simulink model "System_HybridMotorcycle_v2"  (R2013a)
settings: Solver=ode15s  StartTime=0.0  StopTime=500  RelTol=1e-3
values from neighbouring files (symbols this model uses):
  HEV_Param =     [Initialization_v2.mat]
  Speed = SpeedMatrix(i)    [Troubleshooting_Engine_v2_Script1.m]
undefined symbols (not defined in the file or in its folder): Acid, Kt, Kt_Temps, Lead, sigbuilder_block, theta_f, theta_init
libraries: fl_lib x56, nesl_utility x30, sdl_lib x6, LeadAcidBattery_lib x6, simulink x1, electricdrivelib x1, elec_lib x1
(part 1 of 2)
settings Model: Creator=Raymond  LastModifiedBy=Raymond

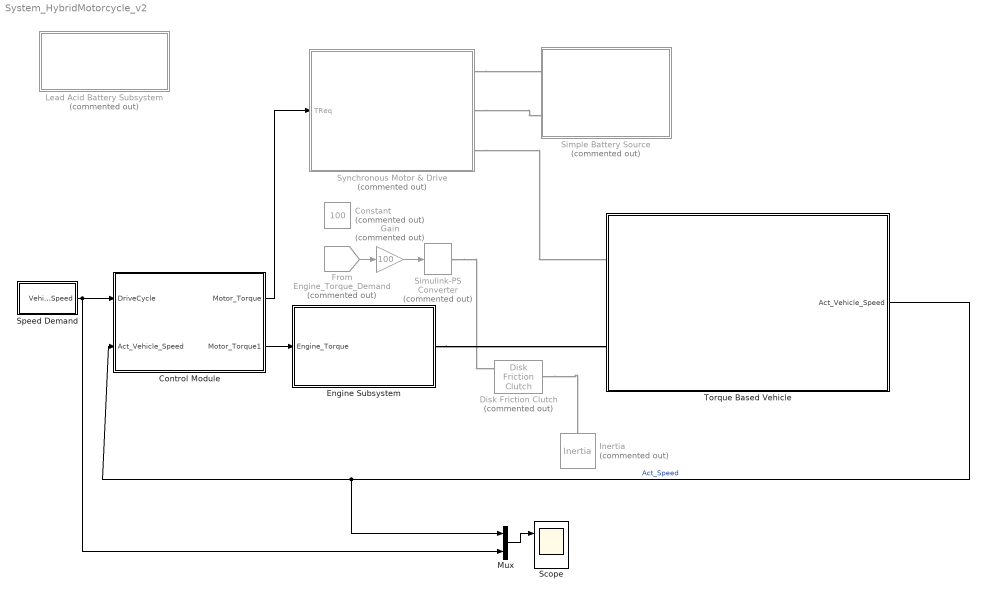
== system System_HybridMotorcycle_v2 ==
  Constant : Constant  Commented=on  Value=100
  Control Module : Subsystem
  Disk Friction Clutch : sdl_lib/Clutches/Disk Friction Clutch  Commented=on  geometry_model=1  r_eff=130 mm  d_o=150 mm  d_i=100 mm  nS=4  piston_area=0.001 m^2  friction_model=1  mu_coulomb=0.3  mu_w_vector=[ 0 0.1 0.2 0.3 0.4 0.5 1 2 5 10 100 1000 ] rad/s  mu_coulomb_vector=[ 0.29 0.28 0.26 0.22 0.21 0.2 0.2 0.19 0.19 0.19 0.19 0.19 ]  mu_interp_method=1  mu_extrap_method=1  mu_static=0.35  d_f=1  w_tol=0.001 rad/s  pressure_min=0.1 Pa  mu_visc=0 N*m/(rad/s)  initial_state_locked=0  LocalVarLogging=[]
  Engine Subsystem : Subsystem
  From : From  Commented=on  GotoTag=Engine_Torque_Demand  TagVisibility=global
  Gain : Gain  Commented=on  Gain=100
  Inertia : fl_lib/Mechanical/Rotational Elements/Inertia  Commented=on  inertia=0.01 kg*m^2  initial_velocity=0 rad/s  t_Log=off  LocalVarNames=|t  LocalVarDescs=|t  LocalVarLogging=0
  Lead Acid Battery Subsystem : Subsystem  Commented=on
  Mux : Mux  Inputs=2
  Scope : Scope  NumInputPorts=2
      settings: YMin=-2.5~0  YMax=50~50  SaveName=ScopeData2
  Simple Battery Source : Subsystem  Commented=on
      mask Display: disp('Simple Battery')
  Simulink-PS Converter : nesl_utility/Simulink-PS Converter  Commented=on  PhysicalDomain=network_engine_domain  SubClassName=ps_input  LeftPortType=input  RightPortType=output  PseudoPeriodic=off  Frequencies=[]  NoiseDistribution=none  NoiseParameters=[]  Unit=1  AffineConversion=off  InputFiltering=off  SimscapeFilterOrder=1  InputFilterTimeConstant=0.001  UdotUserProvided=1
  Speed Demand : Subsystem
      mask Display: disp('DriveCycle')
  Synchronous Motor & Drive : Subsystem  Commented=on
      mask Display:
      | image(imread('HEV_System_Motor_IMAGE.jpg'));
      | port_label('input',1,'T_Req');
      | port_label('RConn',1,'+');
      | port_label('RConn',2,'-');
      | port_label('RConn',3,'Shaft');
  "Torque Based Vehicle " : Subsystem
  wires:
  Speed Demand/1(VehicleSpeed) -> Mux/2, Control Module/1(DriveCycle)
  Control Module/1(Motor_Torque) -> Synchronous Motor & Drive/1(TReq)
  Control Module/2(Motor_Torque1) -> Engine Subsystem/1(Engine_Torque)
  "Torque Based Vehicle "/1(Act_Vehicle_Speed) -> Mux/1, Control Module/2(Act_Vehicle_Speed)  "Act_Speed"
  From/1 -> Gain/1
  Gain/1 -> Simulink-PS Converter/1
  Mux/1 -> Scope/1
  connections:
  Synchronous Motor & Drive/RConn2 -- Simple Battery Source/LConn2
  Synchronous Motor & Drive/RConn1 -- Simple Battery Source/LConn1
  Synchronous Motor & Drive/RConn3 -- "Torque Based Vehicle "/LConn1
  Simulink-PS Converter/RConn1 -- Disk Friction Clutch/LConn1
  Disk Friction Clutch/RConn1 -- Inertia/LConn1
  Engine Subsystem/RConn1 -- "Torque Based Vehicle "/LConn2

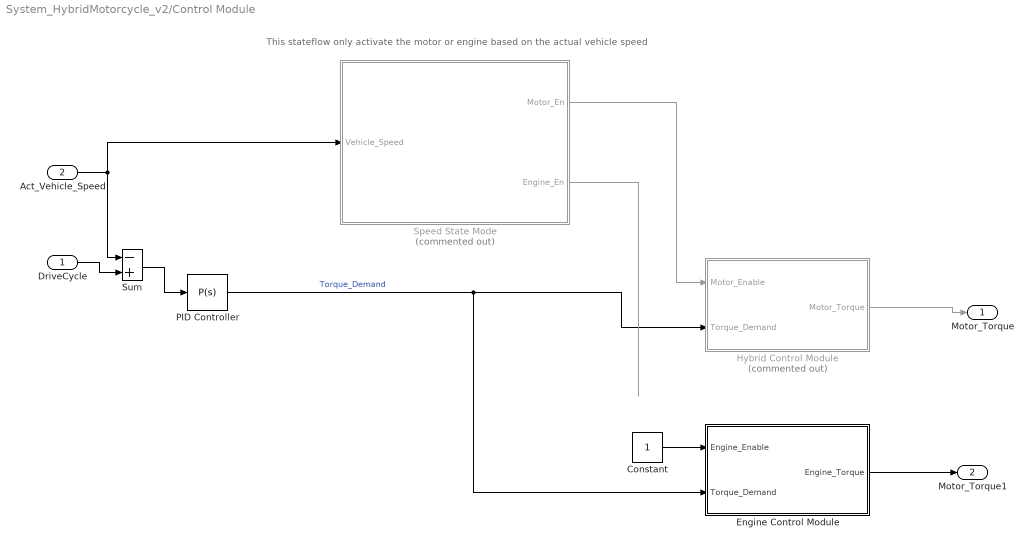
== system System_HybridMotorcycle_v2/Control Module ==
  note: This stateflow only activate the motor or engine
      | based on the actual vehicle speed
  DriveCycle : Inport
  Act_Vehicle_Speed : Inport  Port=2
  Constant : Constant
  Engine Control Module : Subsystem
  Hybrid Control Module : Subsystem  Commented=on
  PID Controller : simulink/Continuous/PID Controller  Controller=P  TimeDomain=Continuous-time  SampleTime=1  IntegratorMethod=Forward Euler  FilterMethod=Forward Euler  Form=Parallel  P=100  I=0  D=0  N=0  InitialConditionSource=internal  InitialConditionForIntegrator=0  InitialConditionForFilter=0  ExternalReset=none  LimitOutput=off  UpperSaturationLimit=inf  LowerSaturationLimit=-inf  LinearizeAsGain=on  AntiWindupMode=none  Kb=1  TrackingMode=off  Kt=1  PParamMin=[]  PParamMax=[]  IParamMin=[]  IParamMax=[]  DParamMin=[]  DParamMax=[]  NParamMin=[]  NParamMax=[]  KbParamMin=[]  KbParamMax=[]  KtParamMin=[]  KtParamMax=[]  POutMin=[]  POutMax=[]  IOutMin=[]  IOutMax=[]  DOutMin=[]  DOutMax=[]  NOutMin=[]  NOutMax=[]  KbOutMin=[]  KbOutMax=[]  KtOutMin=[]  KtOutMax=[]  IntegratorOutMin=[]  IntegratorOutMax=[]  FilterOutMin=[]  FilterOutMax=[]  SumOutMin=[]  SumOutMax=[]  SumI1OutMin=[]  SumI1OutMax=[]  SumI2OutMin=[]  SumI2OutMax=[]  SumI3OutMin=[]  SumI3OutMax=[]  SumDOutMin=[]  SumDOutMax=[]  SaturationOutMin=[]  SaturationOutMax=[]  IntegratorContinuousStateAttributes=''  IntegratorStateMustResolveToSignalObject=off  IntegratorRTWStateStorageClass=Auto  FilterContinuousStateAttributes=''  FilterStateMustResolveToSignalObject=off  FilterRTWStateStorageClass=Auto
  Speed State Mode : Stateflow chart  Commented=on  TreatAsAtomicUnit=on
  Sum : Sum  Inputs=-+
  Motor_Torque : Outport
  Motor_Torque1 : Outport  Port=2
  wires:
  Sum/1 -> PID Controller/1
  PID Controller/1 -> Engine Control Module/2(Torque_Demand), Hybrid Control Module/2(Torque_Demand)  "Torque_Demand"
  Speed State Mode/2(Engine_En) -> ?
  Speed State Mode/1(Motor_En) -> Hybrid Control Module/1(Motor_Enable)
  Hybrid Control Module/1(Motor_Torque) -> Motor_Torque/1
  Engine Control Module/1(Engine_Torque) -> Motor_Torque1/1
  DriveCycle/1 -> Sum/2
  Act_Vehicle_Speed/1 -> Speed State Mode/1(Vehicle_Speed), Sum/1
  Constant/1 -> Engine Control Module/1(Engine_Enable)

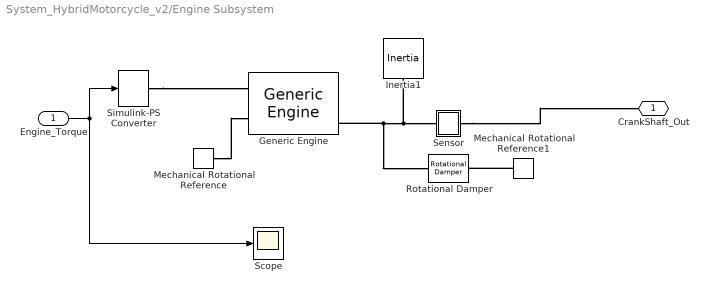
== system System_HybridMotorcycle_v2/Engine Subsystem ==
  Engine_Torque : Inport
  Generic Engine : sdl_lib/Engines/Generic Engine  model_parameterization=1  engine_type=1  P_max=8300 W  w_P_max=8500 rpm  w_max=9000 rpm  w_min=500 rpm  w_tab=[ 500 1000 2e+3 3e+3 4e+3 5e+3 6e+3 7e+3 ] rpm  trq_tab=[ 380 380 380 380 350 280 200 80 ] N*m  pwr_tab=[ 2e+4 4e+4 7.8e+4 1.2e+5 1.45e+5 1.48e+5 1.25e+5 6e+4 ] W  interp_method=1  model_inertia=0  inertia=1 kg*m^2  initial_velocity=800 rpm  model_time_constant=0  time_constant=0.2 s  T0=0  w_thr=100 rpm  idle_speed=1  idle_speed_reference=1000 rpm  tau_controller=1 s  idle_w_thr=1 rpm  fc_model=1  fc_per_rev=25 mg/rev  displaced_volume=400 cm^3  rev_per_cycle=2  fc_w_tab=[ 1000 2e+3 3e+3 4e+3 5e+3 6e+3 ] rpm  fc_trq_tab=[ 0 80 160 200 240 320 360 400 ] N*m  fc_tab=[ 0.5 0.9 1.4 1.6 1.9 2.7 3.4 4.4; 1 1.7 2.7 3.1 3.6 5 6 7.4; 1.4 2.7 4 4.8 5.6 7.5 8.5 10.5; 2 3.6 5.8 6.7 8 10.4 11.7 13.3; 2.5 4.8 7.9 9.4 10.8 14 16.2 18.6; 3.1 6 10.3 11.9 13.8 18.4 22 26.5 ] g/s  bmep_tab=[ 0 250 500 625 750 1000 1.15e+3 1.25e+3 ] kPa  bsfc_tab=[ 410 380 300 280 270 290 320 380; 410 370 290 270 260 270 285 320; 415 380 290 275 265 270 270 300; 420 390 310 290 285 280 280 285; 430 410 340 320 310 300 310 320; 450 430 370 340 330 330 350 380 ] g/hr/kW  fc_interp_method=1  LocalVarLogging=[]
  Inertia1 : fl_lib/Mechanical/Rotational Elements/Inertia  inertia=HEV_Param.ICE.Shaft_Inertia kg*m^2  initial_velocity=0 rad/s  t_Log=off  LocalVarNames=|t  LocalVarDescs=|t  LocalVarLogging=0
  Mechanical Rotational Reference : fl_lib/Mechanical/Rotational Elements/Mechanical Rotational Reference  t_Log=off  LocalVarNames=|t  LocalVarDescs=|t  LocalVarLogging=0
  Mechanical Rotational Reference1 : fl_lib/Mechanical/Rotational Elements/Mechanical Rotational Reference  t_Log=off  LocalVarNames=|t  LocalVarDescs=|t  LocalVarLogging=0
  Rotational Damper : fl_lib/Mechanical/Rotational Elements/Rotational Damper  D=HEV_Param.ICE.Friction N*m/(rad/s)  t_Log=off  w_Log=off  LocalVarNames=|t|w  LocalVarDescs=|t|w  LocalVarLogging=[0 0]
  Scope : Scope
      settings: YMin=-0.05  YMax=1.05  SaveName=ScopeData7
  Sensor : Subsystem
      mask Display: disp('S');
  Simulink-PS Converter : nesl_utility/Simulink-PS Converter  PhysicalDomain=network_engine_domain  SubClassName=ps_input  LeftPortType=input  RightPortType=output  PseudoPeriodic=off  Frequencies=[]  NoiseDistribution=none  NoiseParameters=[]  Unit=N*m  AffineConversion=off  InputFiltering=off  SimscapeFilterOrder=1  InputFilterTimeConstant=0.001  UdotUserProvided=1
  CrankShaft_Out : PMIOPort  Port=1  Side=Right
  wires:
  Engine_Torque/1 -> Simulink-PS Converter/1, Scope/1
  connections:
  Simulink-PS Converter/RConn1 -- Generic Engine/LConn1
  Mechanical Rotational Reference/LConn1 -- Generic Engine/LConn2
  Inertia1/LConn1 -- Rotational Damper/LConn1 -- Generic Engine/RConn3 -- Sensor/LConn1
  Sensor/RConn1 -- CrankShaft_Out/RConn1
  Mechanical Rotational Reference1/LConn1 -- Rotational Damper/RConn1

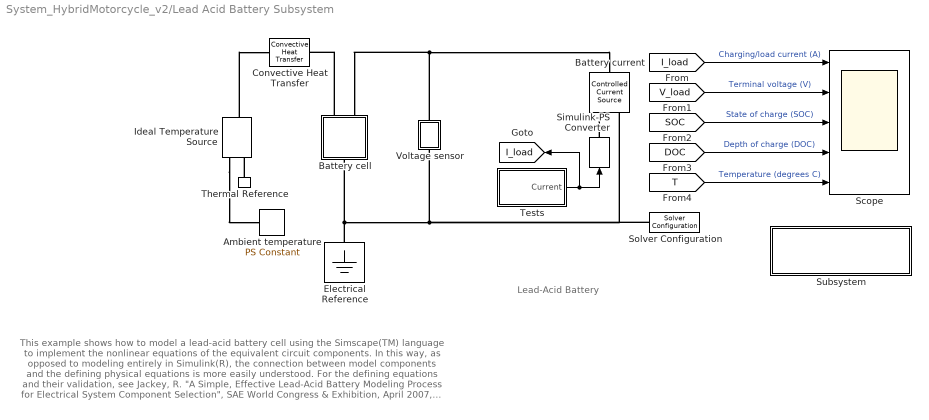
== system System_HybridMotorcycle_v2/Lead Acid Battery Subsystem ==
  note: Lead-Acid Battery
  note: This example shows how to model a lead-acid battery cell using the Simscape(TM) language to implement the nonlinear equations
      | of the equivalent circuit components. In this way, as opposed to modeling entirely in Simulink(R), the connection between model
      | components and the defining physical equations is more easily understood. For the defining equations and their validation,
      | see Jackey, R. "A Simple, Effective Lead-Acid Battery Modeling Process for Electrical System Component Selection",  SAE
      | World Congress & Exhibition, April 2007, ref. 2007-01-0778. In this simulation, initially the battery is discharged at a constant
      | current of 10A. The battery is then recharged at a constant 10A back to the initial state of charge. A simple thermal model is
      | used to model battery temperature. It is assumed that cooling is primarily via convection, and that heating is primarily from
      | battery internal resistance, R2. A standard 12V lead-acid battery can be modeled by connecting six copies of the 2V battery cell
      | block in series.
  Ambient temperature : fl_lib/Physical Signals/Sources/PS Constant  constant=273+25  LocalVarLogging=[]
  Battery cell : Subsystem
      mask Display:
      | image(imread('battery.jpg'))
      | color('red')
      | port_label('LConn',1,'H')
      | port_label('LConn',2,'+')
      | port_label('RConn',1,'-')
  Battery current : fl_lib/Electrical/Electrical Sources/Controlled Current Source  i_Log=off  v_Log=off  LocalVarNames=|current|voltage|power  LocalVarDescs=|Current (A)|Voltage (V)|Power (W)  LocalVarLogging=[0 0 0]
  Convective Heat Transfer : fl_lib/Thermal/Thermal Elements/Convective Heat Transfer  area=Area m^2  heat_tr_coeff=Rtheta W/(m^2 * K)  Q_Log=off  T_Log=off  LocalVarNames=|heat_flow|temperature_diff  LocalVarDescs=|Heat flow (J/s)|Temperature difference (K)  LocalVarLogging=[0 0]
  Electrical Reference : fl_lib/Electrical/Electrical Elements/Electrical Reference  i_Log=off  LocalVarNames=|i  LocalVarDescs=|i  LocalVarLogging=[]
  Ideal Temperature Source : fl_lib/Thermal/Thermal Sources/Ideal Temperature Source  Q_Log=off  T_Log=off  LocalVarNames=|heat_flow|T_differential  LocalVarDescs=|Heat flow rate through the source (J/s)|Temperature differential across the source (K)  LocalVarLogging=[0 0]
  Scope : Scope  NumInputPorts=5
      settings: TimeRange=36000  YMin=-12~1.5~0~0~20  YMax=12~3~1~1~40
  Simulink-PS Converter : nesl_utility/Simulink-PS Converter  PhysicalDomain=network_engine_domain  SubClassName=ps_input  LeftPortType=input  RightPortType=output  PseudoPeriodic=off  Frequencies=[]  NoiseDistribution=none  NoiseParameters=[]  Unit=A  AffineConversion=off  InputFiltering=off  SimscapeFilterOrder=1  InputFilterTimeConstant=.001  UdotUserProvided=0
  Solver Configuration : nesl_utility/Solver Configuration  PhysicalDomain=network_engine_domain  SubClassName=solver  LeftPortType=input  RightPortType=generic  Accelerate=off  Tones=[]  Harmonics=[]  SimulateNoise=off  Profile=off  UseLocalSampling=off  EnableSwitchedLinearOptims=on  FrequencyDomain=off  UseCCode=off  UseNewInitialization=off  DoDC=off  ResidualTolerance=1e-9  UseLocalSolver=off  LocalSolverChoice=NE_BACKWARD_EULER_ADVANCER  LocalSolverSampleTime=.001  DoFixedCost=off  MaxNonlinIter=3  MaxModeIter=2  LinearAlgebra=Sparse  DelaysMemoryBudget=1024
  Subsystem : Subsystem
      settings: OpenFcn=open('LeadAcidBattery_lib')
      mask Display: disp('Open the custom\n library used by the\n Battery cell block')
  Tests : Subsystem  Tag=STV Subsys  LoadFcn=sigbuilder_block('load');  StartFcn=sigbuilder_block('start');  StopFcn=sigbuilder_block('stop');  ClipboardFcn=sigbuilder_block('clipboard');  mask(Sigbuilder block){}
      mask help: Sigbuilder GUI
      mask init:
      | if ~strcmp(get_param(bdroot(gcbh),'SimulationStatus'),'stopped') tuvar = sigbuilder_block('maskInit'); end
      settings: CopyFcn=sigbuilder_block('copy');  DeleteFcn=sigbuilder_block('delete');  ModelCloseFcn=sigbuilder_block('modelClose');  PreSaveFcn=sigbuilder_block('preSave');  PauseFcn=sigbuilder_block('pause')  ContinueFcn=sigbuilder_block('continue')  NameChangeFcn=sigbuilder_block('namechange');  OpenFcn=sigbuilder_block('open',[5.58621 27.931 980.69 471.724 ]);  CloseFcn=sigbuilder_block('close');
      mask Display: plot(0,0,100,100,[10,10,40,40,10],[80,20,20,80,80],[40,10],[50,50], [40,27,10],[65,72,56],[40,25,25,10],[28,28,43,43]);
  Thermal Reference : fl_lib/Thermal/Thermal Elements/Thermal Reference  Q_Log=off  LocalVarNames=|Q  LocalVarDescs=|Q  LocalVarLogging=[]
  Voltage sensor : Subsystem
  tag scope: I_load=global
  wires:
  [V_load] -> Scope/2  "Terminal voltage (V)"
  [SOC] -> Scope/3  "State of charge (SOC)"
  [DOC] -> Scope/4  "Depth of charge (DOC)"
  [T] -> Scope/5  "Temperature (degrees C)"
  [I_load] -> Scope/1  "Charging/load current (A)"
  Tests/1(Current) -> Simulink-PS Converter/1, [I_load]
  connections:
  Electrical Reference/LConn1 -- Battery cell/RConn1 -- Voltage sensor/RConn1 -- Battery current/RConn2 -- Solver Configuration/RConn1
  Voltage sensor/LConn1 -- Battery cell/LConn2 -- Battery current/LConn1
  Thermal Reference/LConn1 -- Ideal Temperature Source/RConn2
  Ideal Temperature Source/LConn1 -- Convective Heat Transfer/LConn1
  Ideal Temperature Source/RConn1 -- Ambient temperature/RConn1
  Battery cell/LConn1 -- Convective Heat Transfer/RConn1
  Simulink-PS Converter/RConn1 -- Battery current/RConn1

== system System_HybridMotorcycle_v2/Simple Battery Source ==
  note: Constant Voltage
  Battery : electricdrivelib/Extra Sources/Battery  Commented=on  BatType=Lead-Acid  ShowDetailedParameters=off  NomV=36  NomQ=30  SOC=100  PresetModel=on  MaxQ=31.25  FullV=39.1974  Dis_rate=6  R=0.012  Normal_OP=9.3083  expZone="[36.6513          0.1]"  Dis_Char=off  current=[6.5 13 32.5]  Units=Ampere-hour  Batt_Tr=30
  Controlled Voltage Source : fl_lib/Electrical/Electrical Sources/Controlled Voltage Source  i_Log=off  v_Log=off  LocalVarNames=|i|v  LocalVarDescs=|i|v  LocalVarLogging=[0 0]
  PS Constant : fl_lib/Physical Signals/Sources/PS Constant  constant=36  LocalVarLogging=[]
  Conn1 : PMIOPort  Port=1  Side=Left
  Conn2 : PMIOPort  Port=2  Side=Left
  connections:
  PS Constant/RConn1 -- Controlled Voltage Source/RConn1
  Controlled Voltage Source/LConn1 -- Conn1/RConn1
  Conn2/RConn1 -- Controlled Voltage Source/RConn2

== system System_HybridMotorcycle_v2/Speed Demand ==
  "10-15 mode " : Subsystem  Tag=STV Subsys  LoadFcn=sigbuilder_block('load');  StartFcn=sigbuilder_block('start');  StopFcn=sigbuilder_block('stop');  ClipboardFcn=sigbuilder_block('clipboard');  mask(Sigbuilder block){}
      mask help: Sigbuilder GUI
      mask init:
      | if ~strcmp(get_param(bdroot(gcbh),'SimulationStatus'),'stopped') tuvar = sigbuilder_block('maskInit'); end
      settings: CopyFcn=sigbuilder_block('copy');  DeleteFcn=sigbuilder_block('delete');  ModelCloseFcn=sigbuilder_block('modelClose');  PreSaveFcn=sigbuilder_block('preSave');  PauseFcn=sigbuilder_block('pause')  ContinueFcn=sigbuilder_block('continue')  NameChangeFcn=sigbuilder_block('namechange');  OpenFcn=sigbuilder_block('open',[5.58621 35.3793 980.69 465.517 ]);  CloseFcn=sigbuilder_block('close');
      mask Display: plot(0,0,100,100,[10,10,40,40,10],[80,20,20,80,80],[40,10],[50,50], [40,27,10],[65,72,56],[40,25,25,10],[28,28,43,43]);
  FTP75 : FromWorkspace  VariableName=[UrbanCycle4.time Vehicle_MaxSpeed_kph/max(UrbanCycle4.SpdKph)*UrbanCycle4.SpdKph]  SampleTime=0
  Multiport Switch : MultiPortSwitch  Inputs=5
  Select Cycle : Constant  Value=4
  Transfer Fcn : TransferFcn  Denominator=[3 1]
  Urban Cycle 1 : FromWorkspace  VariableName=[UrbanCycle1.time UrbanCycle1.SpdKph]  SampleTime=0
  Urban Cycle 2 : FromWorkspace  VariableName=[UrbanCycle2.time UrbanCycle2.SpdKph]  SampleTime=0
  Urban Cycle 3 : FromWorkspace  VariableName=[UrbanCycle3.time UrbanCycle3.SpdKph]  SampleTime=0
  VehicleSpeed : Outport
  wires:
  Urban Cycle 3/1 -> Multiport Switch/4
  Select Cycle/1 -> Multiport Switch/1
  Urban Cycle 2/1 -> Multiport Switch/3
  Urban Cycle 1/1 -> Multiport Switch/2
  FTP75/1 -> Multiport Switch/5
  "10-15 mode "/2(Signal 1) -> Multiport Switch/6
  Transfer Fcn/1 -> VehicleSpeed/1
  Multiport Switch/1 -> Transfer Fcn/1

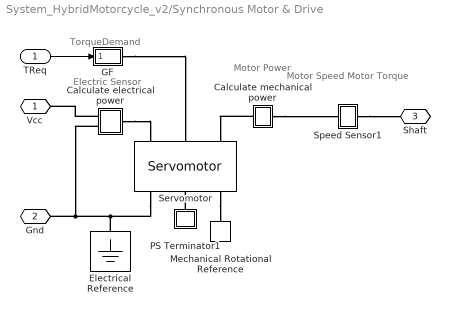
== system System_HybridMotorcycle_v2/Synchronous Motor & Drive ==
  note: Motor Power
  note: TorqueDemand
  note: Electric Sensor
  note: Motor Speed
      | Motor Torque
  TReq : Inport
  Calculate electrical power : Subsystem
      mask Display: disp('S')
  Calculate mechanical power : Subsystem
      mask Display: disp('S')
  Electrical Reference : fl_lib/Electrical/Electrical Elements/Electrical Reference  i_Log=off  LocalVarNames=|i  LocalVarDescs=|i  LocalVarLogging=[]
  GF : Subsystem
      mask Display: disp('GF')
  Mechanical Rotational Reference : fl_lib/Mechanical/Rotational Elements/Mechanical Rotational Reference  t_Log=off  LocalVarNames=|t  LocalVarDescs=|t  LocalVarLogging=[]
  PS Terminator1 : Subsystem
      mask Display:
      | plot([0 0.9],[0.5 0.5]);
      | plot([0.5 0.9],[0.3 0.3]);
      | plot([0.5 0.9],[0.7 0.7]);
      | plot([0.9 0.9],[0.7 0.3]);
  Servomotor : elec_lib/Actuators & Drivers/Rotational Actuators/Servomotor  w_t=[0 2500 3000 3500] rpm  T_t=[15 15 10 0] N*m  Tc=HEV_Param.Motor.TorqueControl_TimeConst s  eff=HEV_Param.Motor.Efficiency  w_eff=2000 rpm  T_eff=200 N*m  Pbase=0 W  Res=0.001 Ohm  J=0 kg*m^2  lam=HEV_Param.Motor.Damping N*m/(rad/s)  speed0=0 rpm  LocalVarLogging=[]  alpha=0.00393 1/K  Tmeas=25 C  thermal_mass=100 J/K  initial_temperature=25 C
  Speed Sensor1 : Subsystem  AncestorBlock=HEV_Electrical_Lib/System Level/Speed Sensor1
      mask Display: disp('S');
  Vcc : PMIOPort  Port=1  Side=Right
  Gnd : PMIOPort  Port=2  Side=Right
  Shaft : PMIOPort  Port=3  Side=Right
  wires:
  TReq/1 -> GF/1(In1)
  connections:
  PS Terminator1/LConn1 -- Servomotor/RConn2
  Servomotor/RConn1 -- Electrical Reference/LConn1 -- Calculate electrical power/LConn2 -- Gnd/RConn1
  GF/RConn1 -- Servomotor/LConn2
  Servomotor/RConn3 -- Mechanical Rotational Reference/LConn1
  Speed Sensor1/RConn1 -- Shaft/RConn1
  Calculate mechanical power/RConn1 -- Speed Sensor1/LConn1
  Calculate mechanical power/LConn1 -- Servomotor/LConn3
  Calculate electrical power/RConn1 -- Servomotor/LConn1
  Calculate electrical power/LConn1 -- Vcc/RConn1

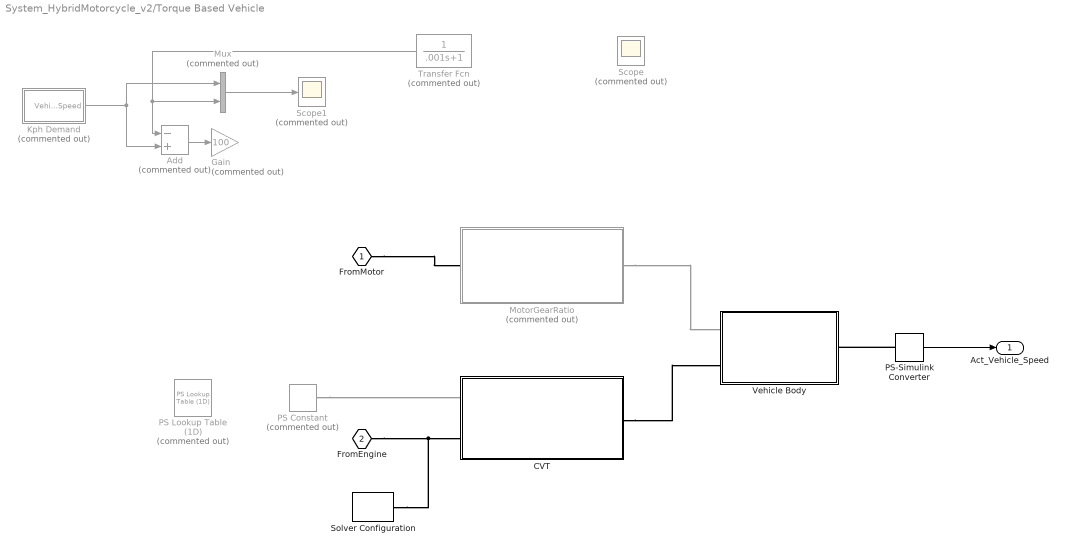
== system System_HybridMotorcycle_v2/Torque Based Vehicle  ==
  Add : Sum  Commented=on  Inputs=-+
  CVT : Subsystem
  Gain : Gain  Commented=on  Gain=100
  Kph Demand : Subsystem  Commented=on
      mask Display: disp('DriveCycle')
  MotorGearRatio : Subsystem  Commented=on
  Mux : Mux  Commented=on  Inputs=2
  PS Constant : fl_lib/Physical Signals/Sources/PS Constant  Commented=on  constant=10  LocalVarLogging=[]
  PS Lookup Table (1D) : fl_lib/Physical Signals/Lookup Tables/PS Lookup Table (1D)  Commented=on  x_t=[1, 2, 3, 4, 5]  y_t=[0, 1, 2, 3, 4]  interp_method=1  extrap_method=1  LocalVarLogging=[]
  PS-Simulink Converter : nesl_utility/PS-Simulink Converter  PhysicalDomain=network_engine_domain  SubClassName=ps_output  LeftPortType=input  RightPortType=output  PseudoPeriodic=off  Frequencies=[]  Unit=mph  AffineConversion=off
  Scope : Scope  Commented=on
      settings: SaveName=ScopeData5
  Scope1 : Scope  Commented=on
      settings: YMax=95
  Solver Configuration : nesl_utility/Solver Configuration  PhysicalDomain=network_engine_domain  SubClassName=solver  LeftPortType=input  RightPortType=generic  Accelerate=off  Tones=[]  Harmonics=[]  SimulateNoise=off  Profile=off  UseLocalSampling=off  EnableSwitchedLinearOptims=on  FrequencyDomain=off  UseCCode=off  UseNewInitialization=off  DoDC=off  ResidualTolerance=1e-09  UseLocalSolver=off  LocalSolverChoice=NE_BACKWARD_EULER_ADVANCER  LocalSolverSampleTime=0.2  DoFixedCost=off  MaxNonlinIter=3  MaxModeIter=2  LinearAlgebra=Sparse  DelaysMemoryBudget=1024
  Transfer Fcn : TransferFcn  Commented=on  Denominator=[.001 1]
  Vehicle Body : Subsystem
  FromMotor : PMIOPort  Port=1  Side=Left
  FromEngine : PMIOPort  Port=2  Side=Left
  Act_Vehicle_Speed : Outport
  wires:
  Kph Demand/1(VehicleSpeed) -> Mux/1, Add/2
  Add/1 -> Gain/1
  Transfer Fcn/1 -> Mux/2, Add/1
  Mux/1 -> Scope1/1
  PS-Simulink Converter/1 -> Act_Vehicle_Speed/1
  connections:
  FromMotor/RConn1 -- MotorGearRatio/LConn1
  PS-Simulink Converter/LConn1 -- Vehicle Body/RConn1
  MotorGearRatio/RConn1 -- Vehicle Body/LConn1
  FromEngine/RConn1 -- Solver Configuration/RConn1 -- CVT/LConn2
  CVT/RConn1 -- Vehicle Body/LConn2
  PS Constant/RConn1 -- CVT/LConn1

== system System_HybridMotorcycle_v2/Control Module/Engine Control Module ==
  Engine_Enable : Inport
  Torque_Demand : Inport  Port=2
  Engine Off : Constant  Value=0
  Switch : Switch  Threshold=0.5
  Engine_Torque : Outport
  tag scope: Engine_Torque_Demand=global
  wires:
  Engine Off/1 -> Switch/3
  Switch/1 -> [Engine_Torque_Demand], Engine_Torque/1
  Engine_Enable/1 -> Switch/2
  Torque_Demand/1 -> Switch/1

== system System_HybridMotorcycle_v2/Control Module/Hybrid Control Module ==
  Motor_Enable : Inport
  Torque_Demand : Inport  Port=2
  Motor Off : Constant  Value=0
  Switch : Switch  Threshold=0.5
  Motor_Torque : Outport
  wires:
  Motor_Enable/1 -> Switch/2
  Torque_Demand/1 -> Switch/1
  Motor Off/1 -> Switch/3
  Switch/1 -> Motor_Torque/1

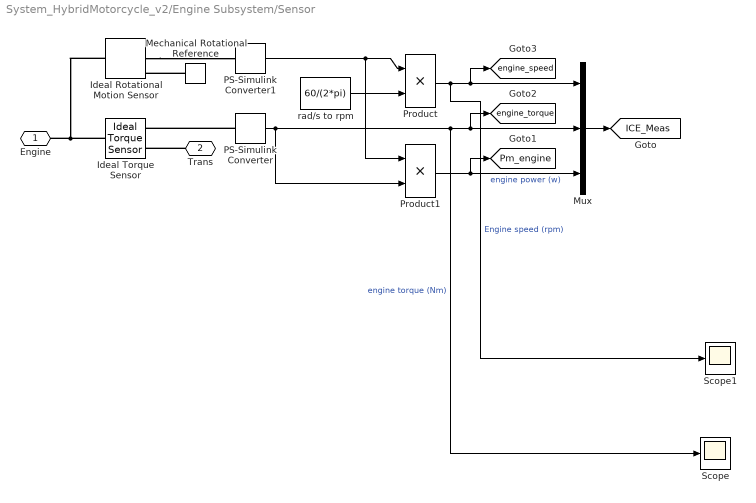
== system System_HybridMotorcycle_v2/Engine Subsystem/Sensor ==
  Ideal Rotational Motion Sensor : fl_lib/Mechanical/Mechanical Sensors/Ideal Rotational Motion Sensor  offset=0 rad  w_Log=off  t_Log=off  phi_Log=off  LocalVarNames=|w|t|phi  LocalVarDescs=|w|t|phi  LocalVarLogging=[0 0 0]
  Ideal Torque Sensor : fl_lib/Mechanical/Mechanical Sensors/Ideal Torque Sensor  w_Log=off  t_Log=off  LocalVarNames=|w|t  LocalVarDescs=|w|t  LocalVarLogging=[0 0]
  Mechanical Rotational Reference : fl_lib/Mechanical/Rotational Elements/Mechanical Rotational Reference  t_Log=off  LocalVarNames=|t  LocalVarDescs=|t  LocalVarLogging=0
  Mux : Mux  Inputs=3
  PS-Simulink Converter : nesl_utility/PS-Simulink Converter  PhysicalDomain=network_engine_domain  SubClassName=ps_output  LeftPortType=input  RightPortType=output  PseudoPeriodic=off  Frequencies=[]  Unit=N*m  AffineConversion=off
  PS-Simulink Converter1 : nesl_utility/PS-Simulink Converter  PhysicalDomain=network_engine_domain  SubClassName=ps_output  LeftPortType=input  RightPortType=output  PseudoPeriodic=off  Frequencies=[]  Unit=rad/s  AffineConversion=off
  Product : Product  RndMeth=Zero
  Product1 : Product  RndMeth=Zero
  Scope : Scope
      settings: YMin=-0.0175  YMax=0.0175  SaveName=ScopeData3
  Scope1 : Scope
      settings: YMin=-2.5e-14  YMax=4.5e-13  SaveName=ScopeData6
  rad/s to rpm : Constant  Value=60/(2*pi)
  Engine : PMIOPort  Port=1  Side=Left
  Trans : PMIOPort  Port=2  Side=Right
  tag scope: ICE_Meas=global, Pm_engine=global, engine_speed=global, engine_torque=global
  wires:
  PS-Simulink Converter/1 -> Product1/2, Scope/1, Mux/2, [engine_torque]  "engine torque (Nm)"
  Product1/1 -> Mux/3, [Pm_engine]  "engine power (w)"
  Product/1 -> Scope1/1, Mux/1, [engine_speed]  "Engine speed (rpm)"
  PS-Simulink Converter1/1 -> Product/1, Product1/1
  rad/s to rpm/1 -> Product/2
  Mux/1 -> [ICE_Meas]
  connections:
  Ideal Torque Sensor/LConn1 -- Engine/RConn1 -- Ideal Rotational Motion Sensor/LConn1
  Trans/RConn1 -- Ideal Torque Sensor/RConn1
  PS-Simulink Converter/LConn1 -- Ideal Torque Sensor/RConn2
  Ideal Rotational Motion Sensor/RConn2 -- PS-Simulink Converter1/LConn1
  Mechanical Rotational Reference/LConn1 -- Ideal Rotational Motion Sensor/RConn1

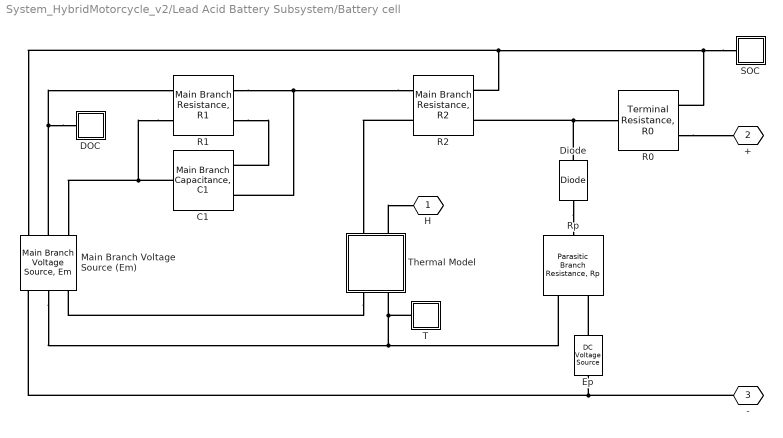
== system System_HybridMotorcycle_v2/Lead Acid Battery Subsystem/Battery cell ==
  " DOC " : Subsystem
  " SOC " : Subsystem
  C1 : LeadAcidBattery_lib/Main Branch Capacitance, C1  Tau1=Tau1 s  Cmin=1e-5 F  i_Log=off  v_Log=off  Q_Log=off  LocalVarNames=|i|v|Q  LocalVarDescs=|Current through variable|Voltage across variable|Charge variable  LocalVarLogging=[0 0 0]
  Diode : fl_lib/Electrical/Electrical Elements/Diode  Vf=0.6 V  Ron=0.3 Ohm  Goff=1e-08 1/Ohm  i_Log=off  v_Log=off  LocalVarNames=|current|voltage|power  LocalVarDescs=|Diode current (A)|Voltage across diode (V)|Power (W)  LocalVarLogging=[0 0 0]
  Ep : fl_lib/Electrical/Electrical Sources/DC Voltage Source  v0=Ep V  i_Log=off  v_Log=off  LocalVarNames=|current|voltage|power  LocalVarDescs=|Current (A)|Voltage (V)|Power (W)  LocalVarLogging=[0 0 0]
  Main Branch Voltage Source (Em) : LeadAcidBattery_lib/Main Branch Voltage Source, Em  Em0=Emo V  Ke=Ke V/K  Kc=Kc  C0=Costar s*A  Istar=Istar A  delta=delta  Tau1=Tau1 s  Qinit=Qe_init s*A  i_Log=off  v_Log=off  Iavg_Log=off  Qe_Log=off  LocalVarNames=|i|v|cap_u|cap_t|Q|Iavg  LocalVarDescs=|Current through variable|Voltage across variable|usable battery capacity|total battery capacity|battery charge|average current given by (I/(Ts+1))  LocalVarLogging=[0 0 0 0 0 0]
  R0 : LeadAcidBattery_lib/Terminal Resistance, R0  R00=Roo Ohm  A0=Ao  i_Log=off  v_Log=off  LocalVarNames=|i|v  LocalVarDescs=|Current through variable|Voltage across variable  LocalVarLogging=[0 0]
  R1 : LeadAcidBattery_lib/Main Branch Resistance, R1  R10=R10 Ohm  DOC_min=1e-006  i_Log=off  v_Log=off  LocalVarNames=|i|v  LocalVarDescs=|Current through variable|Voltage across variable  LocalVarLogging=[0 0]
  R2 : LeadAcidBattery_lib/Main Branch Resistance, R2  R20=R20 Ohm  A21=A21  A22=A22  Istar=Istar A  i_Log=off  v_Log=off  LocalVarNames=|i|v  LocalVarDescs=|Current through variable|Voltage across variable  LocalVarLogging=[0 0]
  Rp : LeadAcidBattery_lib/Parasitic Branch Resistance, Rp  Gp0=Gpo 1/Ohm  Vp0=Vpo V  Ap=Ap  Tf=theta_f C  i_Log=off  v_Log=off  LocalVarNames=|i|v|Vavg  LocalVarDescs=|Current through variable|Voltage across variable|average voltage given by (V/(Ts+1))  LocalVarLogging=[0 0 0]
  T : Subsystem
  Thermal Model : Subsystem
  H : PMIOPort  Tag=PMCPort  Port=1  Side=Left
  + : PMIOPort  Tag=PMCPort  Port=2  Side=Left
  - : PMIOPort  Tag=PMCPort  Port=3  Side=Right
  connections:
  Thermal Model/RConn2 -- T/LConn1 -- Rp/RConn1 -- Main Branch Voltage Source (Em)/RConn2
  R0/LConn2 -- +/RConn1
  " DOC "/LConn1 -- R1/RConn1 -- Main Branch Voltage Source (Em)/LConn2
  R1/RConn2 -- C1/RConn1 -- Main Branch Voltage Source (Em)/LConn3
  R2/RConn1 -- C1/LConn2 -- R1/LConn1
  R1/LConn2 -- C1/LConn1
  " SOC "/LConn1 -- R0/LConn1 -- Main Branch Voltage Source (Em)/LConn1 -- R2/LConn1
  Thermal Model/LConn2 -- H/RConn1
  Ep/LConn1 -- Rp/RConn2
  Diode/RConn1 -- Rp/LConn1
  Thermal Model/RConn1 -- Main Branch Voltage Source (Em)/RConn3
  Main Branch Voltage Source (Em)/RConn1 -- Ep/RConn1 -- -/RConn1
  R2/RConn2 -- Thermal Model/LConn1
  R2/LConn2 -- R0/RConn1 -- Diode/LConn1

== system System_HybridMotorcycle_v2/Lead Acid Battery Subsystem/Subsystem ==

== system System_HybridMotorcycle_v2/Lead Acid Battery Subsystem/Tests ==
  Demux : Demux  Tag=STV Demux  Outputs=1
  FromWs : FromWorkspace  Tag=STV FromWs  VariableName=tuvar  SampleTime=0
      SigBuilderData=|
      | common.afterFinalStr = 'Extrapolate'
      | common.sampleTime = 0
      | dataSet(1).timeRange = [0 36000]
      | dataSet(1).name = 'Dynamic'
      | dataSet(2).timeRange = [0 36000]
      | dataSet(2).name = 'Charge Cycle'
      | dataSet(3).timeRange = [0 36000]
      | dataSet(3).name = 'Square'
      | sbobj.Groups(1).Name = 'Dynamic'
      | sbobj.Groups(1).Signals.Name = 'Current'
      | sbobj.Groups(1).Signals.XData = [0 60 120 180 240 300 360 420 480 540 600 660 ... (607 elements, 1x607)]
      | sbobj.Groups(1).Signals.YData = [-4.32564811528 -16.6558437824 1.25332306475 2.87676420359 -11.4647135068 11.9091546564 11.8916420165 -0.376332765933 3.27292361409 1.74639142821 -1.86708577681 7.25790548293 ... (607 elements, 1x607)]
      | sbobj.Groups(2).Name = 'Charge Cycle'
      | sbobj.Groups(2).Signals.Name = 'Current'
      | sbobj.Groups(2).Signals.XData = [0 1000 1000 12630 12630 18400 28090 35015 36000]
      | sbobj.Groups(2).Signals.YData = [0 0 -10 -10 0 10 10 0 0]
      | sbobj.Groups(3).Name = 'Square'
      | sbobj.Groups(3).Signals.Name = 'Current'
      | sbobj.Groups(3).Signals.XData = [0 3600 3600 5400 5400 7200 7200 9000 9000 10800 10800 12600 12600 14400 14400 16200 16200 18000 18000 19800 19800 21600 21600 23400 23400 25200 25200 27000 27000 28800 28800 30600 30600 32400 32400 34200 34200 36000]
      | sbobj.Groups(3).Signals.YData = [-20 -20 0 0 20 20 -20 -20 20 20 -20 -20 20 20 -20 -20 20 20 -20 -20 20 20 -20 -20 20 20 -20 -20 20 20 -20 -20 20 20 -20 -20 20 20]
  Current : Outport  Tag=STV Outport
  wires:
  Demux/1 -> Current/1
  FromWs/1 -> Demux/1

== system System_HybridMotorcycle_v2/Lead Acid Battery Subsystem/Voltage sensor ==
  PS-Simulink Converter : nesl_utility/PS-Simulink Converter  PhysicalDomain=network_engine_domain  SubClassName=ps_output  LeftPortType=input  RightPortType=output  PseudoPeriodic=off  Frequencies=[]  Unit=V  AffineConversion=off
  Voltage Sensor : fl_lib/Electrical/Electrical Sensors/Voltage Sensor  i1_Log=off  v1_Log=off  LocalVarNames=|i1|v1  LocalVarDescs=|i1|v1  LocalVarLogging=[]
  + : PMIOPort  Port=1  Side=Left
  - : PMIOPort  Port=2  Side=Right
  tag scope: V_load=global
  wires:
  PS-Simulink Converter/1 -> [V_load]
  connections:
  Voltage Sensor/RConn1 -- PS-Simulink Converter/LConn1
  +/RConn1 -- Voltage Sensor/LConn1
  -/RConn1 -- Voltage Sensor/RConn2

== system System_HybridMotorcycle_v2/Speed Demand/10-15 mode  ==
  Demux : Demux  Tag=STV Demux  Outputs=2
  FromWs : FromWorkspace  Tag=STV FromWs  VariableName=tuvar  SampleTime=0
      SigBuilderData=|
      | common.afterFinalStr = 'Extrapolate'
      | common.sampleTime = '0'
      | dataSet.timeRange = [0 660]
      | dataSet.name = '10-15 Mode Cycle'
      | sbobj.Groups.Name = '10-15 Mode Cycle'
      | sbobj.Groups.Signals(1).Name = 'Target speed'
      | sbobj.Groups.Signals(1).XData = [0 44 51 73 73 89 103 118 128 130 142 152 159 179 186 201 208 224 238 253 263 265 277 287 294 314 321 336 343 359 373 388 398 400 412 422 429 494 512 524 528 532 548 558 569 579 589 593 615 620 640 650 660]
      | sbobj.Groups.Signals(1).YData = [0 0 10 10 0 0 40 40 20 20 40 20 0 0 20 20 0 0 40 40 20 20 40 20 0 0 20 20 0 0 40 40 20 20 40 20 0 0 50 50 40 40 60 60 70 70 50 50 70 70 30 0 0]
      | sbobj.Groups.Signals(2).Name = 'Signal 1'
      | sbobj.Groups.Signals(2).XData = [0 20 120 120 220 220 320 320 420 420 520 520 620 650 660]
      | sbobj.Groups.Signals(2).YData = [0 10 10 20 20 30 30 40 39.8 50 50 60 60 0.5 0]
  Target speed : Outport  Tag=STV Outport
  Signal 1 : Outport  Tag=STV Outport  Port=2
  wires:
  FromWs/1 -> Demux/1
  Demux/1 -> Target speed/1
  Demux/2 -> Signal 1/1

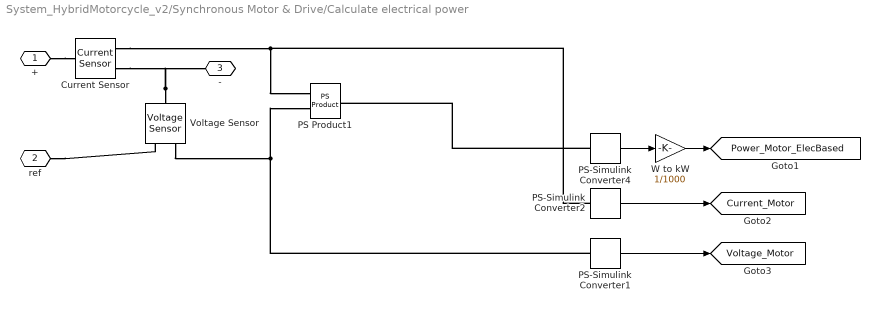
== system System_HybridMotorcycle_v2/Synchronous Motor & Drive/Calculate electrical power ==
  Current Sensor : fl_lib/Electrical/Electrical Sensors/Current Sensor  i1_Log=off  v1_Log=off  LocalVarNames=|i1|v1  LocalVarDescs=|i1|v1  LocalVarLogging=[]
  PS Product1 : fl_lib/Physical Signals/Functions/PS Product  LocalVarLogging=[]
  PS-Simulink Converter1 : nesl_utility/PS-Simulink Converter  PhysicalDomain=network_engine_domain  SubClassName=ps_output  LeftPortType=input  RightPortType=output  PseudoPeriodic=off  Frequencies=[]  Unit=V  AffineConversion=off
  PS-Simulink Converter2 : nesl_utility/PS-Simulink Converter  PhysicalDomain=network_engine_domain  SubClassName=ps_output  LeftPortType=input  RightPortType=output  PseudoPeriodic=off  Frequencies=[]  Unit=A  AffineConversion=off
  PS-Simulink Converter4 : nesl_utility/PS-Simulink Converter  PhysicalDomain=network_engine_domain  SubClassName=ps_output  LeftPortType=input  RightPortType=output  PseudoPeriodic=off  Frequencies=[]  Unit=W  AffineConversion=off
  Voltage Sensor : fl_lib/Electrical/Electrical Sensors/Voltage Sensor  i1_Log=off  v1_Log=off  LocalVarNames=|i1|v1  LocalVarDescs=|i1|v1  LocalVarLogging=[]
  W to kW : Gain  Gain=1/1000
  + : PMIOPort  Port=1  Side=Left
  ref : PMIOPort  Port=2  Side=Left
  - : PMIOPort  Port=3  Side=Right
  tag scope: Current_Motor=global, Power_Motor_ElecBased=global, Voltage_Motor=global
  wires:
  PS-Simulink Converter4/1 -> W to kW/1
  W to kW/1 -> [Power_Motor_ElecBased]
  PS-Simulink Converter1/1 -> [Voltage_Motor]
  PS-Simulink Converter2/1 -> [Current_Motor]
  connections:
  ref/RConn1 -- Voltage Sensor/RConn2
  +/RConn1 -- Current Sensor/LConn1
  PS-Simulink Converter4/LConn1 -- PS Product1/RConn1
  Voltage Sensor/RConn1 -- PS-Simulink Converter1/LConn1 -- PS Product1/LConn2
  Voltage Sensor/LConn1 -- Current Sensor/RConn2 -- -/RConn1
  Current Sensor/RConn1 -- PS-Simulink Converter2/LConn1 -- PS Product1/LConn1

== system System_HybridMotorcycle_v2/Synchronous Motor & Drive/Calculate mechanical power ==
  Ideal Rotational Motion Sensor : fl_lib/Mechanical/Mechanical Sensors/Ideal Rotational Motion Sensor  offset=0 rad  w_Log=off  t_Log=off  phi_Log=off  LocalVarNames=|w|t|phi  LocalVarDescs=|w|t|phi  LocalVarLogging=[]
  Mechanical Rotational Reference1 : fl_lib/Mechanical/Rotational Elements/Mechanical Rotational Reference  t_Log=off  LocalVarNames=|t  LocalVarDescs=|t  LocalVarLogging=[]
  PS Product : fl_lib/Physical Signals/Functions/PS Product  LocalVarLogging=[]
  PS-Simulink Converter3 : nesl_utility/PS-Simulink Converter  PhysicalDomain=network_engine_domain  SubClassName=ps_output  LeftPortType=input  RightPortType=output  PseudoPeriodic=off  Frequencies=[]  Unit=W  AffineConversion=off
  Torque Sensor : fl_lib/Mechanical/Mechanical Sensors/Ideal Torque Sensor  w_Log=off  t_Log=off  LocalVarNames=|w|t  LocalVarDescs=|w|t  LocalVarLogging=[]
  W to kW : Gain  Gain=1/1000
  C : PMIOPort  Port=1  Side=Right
  R : PMIOPort  Port=2  Side=Left
  tag scope: Power_Motor_MechBased=global
  wires:
  W to kW/1 -> [Power_Motor_MechBased]
  PS-Simulink Converter3/1 -> W to kW/1
  connections:
  Mechanical Rotational Reference1/LConn1 -- Ideal Rotational Motion Sensor/RConn1
  Ideal Rotational Motion Sensor/RConn2 -- PS Product/LConn2
  Torque Sensor/RConn2 -- PS Product/LConn1
  PS Product/RConn1 -- PS-Simulink Converter3/LConn1
  Ideal Rotational Motion Sensor/LConn1 -- Torque Sensor/LConn1 -- R/RConn1
  C/RConn1 -- Torque Sensor/RConn1

== system System_HybridMotorcycle_v2/Synchronous Motor & Drive/GF ==
  In1 : Inport
  Simulink-PS Converter : nesl_utility/Simulink-PS Converter  PhysicalDomain=network_engine_domain  SubClassName=ps_input  LeftPortType=input  RightPortType=output  PseudoPeriodic=off  Frequencies=[]  NoiseDistribution=none  NoiseParameters=[]  Unit=N*m  AffineConversion=off  InputFiltering=on  SimscapeFilterOrder=1  InputFilterTimeConstant=.001  UdotUserProvided=1
  Conn1 : PMIOPort  Port=1  Side=Right
  tag scope: Mot_TReq_SYS=global
  wires:
  In1/1 -> Simulink-PS Converter/1, [Mot_TReq_SYS]
  connections:
  Simulink-PS Converter/RConn1 -- Conn1/RConn1

== system System_HybridMotorcycle_v2/Synchronous Motor & Drive/PS Terminator1 ==
  PS-Simulink Converter 2 : nesl_utility/PS-Simulink Converter  PhysicalDomain=network_engine_domain  SubClassName=ps_output  LeftPortType=input  RightPortType=output  PseudoPeriodic=off  Frequencies=[]  Unit=rpm  AffineConversion=off
  Terminator : Terminator
  R : PMIOPort  Port=1  Side=Left
  wires:
  PS-Simulink Converter 2/1 -> Terminator/1
  connections:
  R/RConn1 -- PS-Simulink Converter 2/LConn1

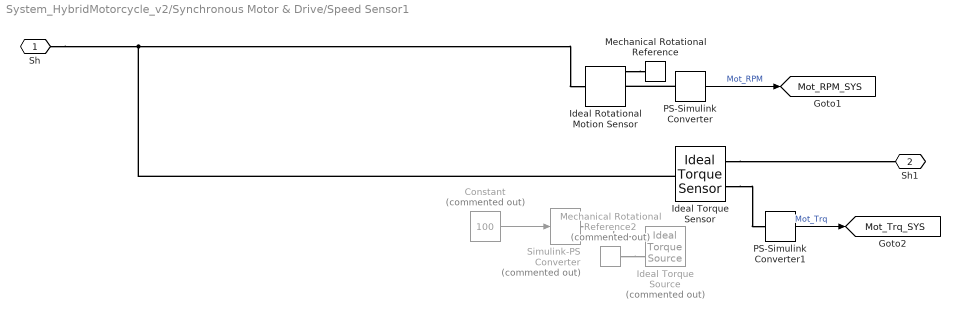
== system System_HybridMotorcycle_v2/Synchronous Motor & Drive/Speed Sensor1 ==
  Constant : Constant  Commented=on  Value=100
  Ideal Rotational Motion Sensor : fl_lib/Mechanical/Mechanical Sensors/Ideal Rotational Motion Sensor  offset=0 rad  w_Log=off  t_Log=off  phi_Log=off  LocalVarNames=|w|t|phi  LocalVarDescs=|w|t|phi  LocalVarLogging=[0 0 0]
  Ideal Torque Sensor : fl_lib/Mechanical/Mechanical Sensors/Ideal Torque Sensor  w_Log=off  t_Log=off  LocalVarNames=|w|t  LocalVarDescs=|w|t  LocalVarLogging=[0 0]
  Ideal Torque Source : fl_lib/Mechanical/Mechanical Sources/Ideal Torque Source  Commented=on  w_Log=off  t_Log=off  LocalVarNames=|w|t  LocalVarDescs=|w|t  LocalVarLogging=[0 0]
  Mechanical Rotational Reference : fl_lib/Mechanical/Rotational Elements/Mechanical Rotational Reference  t_Log=off  LocalVarNames=|t  LocalVarDescs=|t  LocalVarLogging=0
  Mechanical Rotational Reference2 : fl_lib/Mechanical/Rotational Elements/Mechanical Rotational Reference  Commented=on  t_Log=off  LocalVarNames=|t  LocalVarDescs=|t  LocalVarLogging=0
  PS-Simulink Converter : nesl_utility/PS-Simulink Converter  PhysicalDomain=network_engine_domain  SubClassName=ps_output  LeftPortType=input  RightPortType=output  PseudoPeriodic=off  Frequencies=[]  Unit=rpm  AffineConversion=off
  PS-Simulink Converter1 : nesl_utility/PS-Simulink Converter  PhysicalDomain=network_engine_domain  SubClassName=ps_output  LeftPortType=input  RightPortType=output  PseudoPeriodic=off  Frequencies=[]  Unit=N*m  AffineConversion=off
  Simulink-PS Converter : nesl_utility/Simulink-PS Converter  Commented=on  PhysicalDomain=network_engine_domain  SubClassName=ps_input  LeftPortType=input  RightPortType=output  PseudoPeriodic=off  Frequencies=[]  NoiseDistribution=none  NoiseParameters=[]  Unit=1  AffineConversion=off  InputFiltering=off  SimscapeFilterOrder=1  InputFilterTimeConstant=0.001  UdotUserProvided=1
  Sh : PMIOPort  Port=1  Side=Left
  Sh1 : PMIOPort  Port=2  Side=Right
  tag scope: Mot_RPM_SYS=global, Mot_Trq_SYS=global
  wires:
  PS-Simulink Converter/1 -> [Mot_RPM_SYS]  "Mot_RPM"
  PS-Simulink Converter1/1 -> [Mot_Trq_SYS]  "Mot_Trq"
  Constant/1 -> Simulink-PS Converter/1
  connections:
  PS-Simulink Converter/LConn1 -- Ideal Rotational Motion Sensor/RConn2
  Ideal Torque Sensor/LConn1 -- Ideal Rotational Motion Sensor/LConn1 -- Sh/RConn1
  Ideal Rotational Motion Sensor/RConn1 -- Mechanical Rotational Reference/LConn1
  Ideal Torque Sensor/RConn2 -- PS-Simulink Converter1/LConn1
  Mechanical Rotational Reference2/LConn1 -- Ideal Torque Source/RConn2
  Simulink-PS Converter/RConn1 -- Ideal Torque Source/RConn1
  Ideal Torque Sensor/RConn1 -- Sh1/RConn1

== system System_HybridMotorcycle_v2/Torque Based Vehicle /CVT ==
  From : From  Commented=on  GotoTag=Engine_Torque_Demand  TagVisibility=global
  Simulink-PS Converter : nesl_utility/Simulink-PS Converter  Commented=on  PhysicalDomain=network_engine_domain  SubClassName=ps_input  LeftPortType=input  RightPortType=output  PseudoPeriodic=off  Frequencies=[]  NoiseDistribution=none  NoiseParameters=[]  Unit=1  AffineConversion=off  InputFiltering=off  SimscapeFilterOrder=1  InputFilterTimeConstant=0.001  UdotUserProvided=1
  Variable Ratio Transmission : sdl_lib/Couplings & Drives/Variable Ratio Transmission  Commented=on  rotation_direction=1  kp=3e+5 N*m/rad  kv=0.05 N*m/(rad/s)  initial_torque=0 N*m  losses_model=1  efficiency=0.8  mu_visc=[ 0 0 ] N*m/(rad/s)  w_thr=0.01 rad/s  LocalVarLogging=[]
  VariableRatio : PMIOPort  Port=1  Side=Left
  ToRearWheel : PMIOPort  Port=2  Side=Right
  ToEngine : PMIOPort  Port=3  Side=Left
  wires:
  From/1 -> Simulink-PS Converter/1
  connections:
  ToEngine/RConn1 -- ToRearWheel/RConn1
  Variable Ratio Transmission/LConn1 -- VariableRatio/RConn1

== system System_HybridMotorcycle_v2/Torque Based Vehicle /Kph Demand ==
  "10-15 mode " : Subsystem  Tag=STV Subsys  LoadFcn=sigbuilder_block('load');  StartFcn=sigbuilder_block('start');  StopFcn=sigbuilder_block('stop');  ClipboardFcn=sigbuilder_block('clipboard');  mask(Sigbuilder block){}
      mask help: Sigbuilder GUI
      mask init:
      | if ~strcmp(get_param(bdroot(gcbh),'SimulationStatus'),'stopped') tuvar = sigbuilder_block('maskInit'); end
      settings: CopyFcn=sigbuilder_block('copy');  DeleteFcn=sigbuilder_block('delete');  ModelCloseFcn=sigbuilder_block('modelClose');  PreSaveFcn=sigbuilder_block('preSave');  PauseFcn=sigbuilder_block('pause')  ContinueFcn=sigbuilder_block('continue')  NameChangeFcn=sigbuilder_block('namechange');  OpenFcn=sigbuilder_block('open',[5.58621 35.3793 980.69 465.517 ]);  CloseFcn=sigbuilder_block('close');
      mask Display: plot(0,0,100,100,[10,10,40,40,10],[80,20,20,80,80],[40,10],[50,50], [40,27,10],[65,72,56],[40,25,25,10],[28,28,43,43]);
  FTP75 : FromWorkspace  VariableName=[UrbanCycle4.time Vehicle_MaxSpeed_kph/max(UrbanCycle4.SpdKph)*UrbanCycle4.SpdKph]  SampleTime=0
  Multiport Switch : MultiPortSwitch  Inputs=5
  Select Cycle : Constant  Value=4
  Transfer Fcn : TransferFcn  Denominator=[3 1]
  Urban Cycle 1 : FromWorkspace  VariableName=[UrbanCycle1.time UrbanCycle1.SpdKph]  SampleTime=0
  Urban Cycle 2 : FromWorkspace  VariableName=[UrbanCycle2.time UrbanCycle2.SpdKph]  SampleTime=0
  Urban Cycle 3 : FromWorkspace  VariableName=[UrbanCycle3.time UrbanCycle3.SpdKph]  SampleTime=0
  VehicleSpeed : Outport
  wires:
  Urban Cycle 3/1 -> Multiport Switch/4
  Select Cycle/1 -> Multiport Switch/1
  Urban Cycle 2/1 -> Multiport Switch/3
  Urban Cycle 1/1 -> Multiport Switch/2
  FTP75/1 -> Multiport Switch/5
  "10-15 mode "/2(Signal 1) -> Multiport Switch/6
  Transfer Fcn/1 -> VehicleSpeed/1
  Multiport Switch/1 -> Transfer Fcn/1

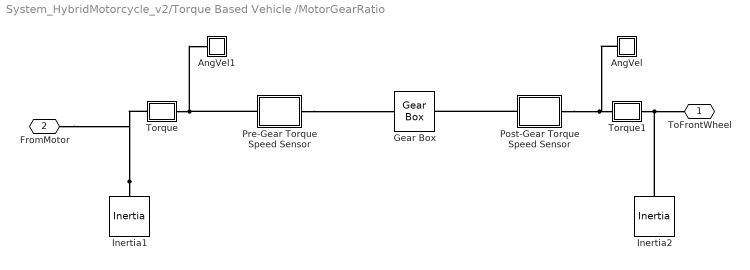
== system System_HybridMotorcycle_v2/Torque Based Vehicle /MotorGearRatio ==
  AngVel : Subsystem  InitFcn=|
      | unit=get_param([gcb '/PS-S'],'Unit');
      | set_param(gcb, 'AttributesFormatString', strcat('[', unit,']'));
      mask help: Simscape Probe
      settings: AttributesFormatString=[rpm]
      settings: CopyFcn=|
      | set_param(gcb,'LinkStatus','inactive')
      | set_param(gcb,'LinkStatus','none')
      | set_param([gcb '/Goto'],'GotoTag', [get(gcbh,'name')])
      | 
      | set_param([gcb '/From'],'GotoTag', [get(gcbh,'name')])
      settings: NameChangeFcn=|
      | set_param([gcb '/Goto'],'GotoTag', [get(gcbh,'name')])
      | 
      | set_param([gcb '/From'],'GotoTag', [get(gcbh,'name')])
      settings: OpenFcn=|
      | open_system([gcb '/ang_vel']);
      | close_system(gcb);                    hh=findobj(allchild(0),'name','ang_vel');
      | ha=findobj(hh(1),'type','axes');
      | set(get(ha,'title'),'string',get(gcbh,'name'));
      | clear hh ha;
      mask Display: port_label('LConn', 1,'W');
  AngVel1 : Subsystem  InitFcn=|
      | unit=get_param([gcb '/PS-S'],'Unit');
      | set_param(gcb, 'AttributesFormatString', strcat('[', unit,']'));
      mask help: Simscape Probe
      settings: AttributesFormatString=[rpm]
      settings: CopyFcn=|
      | set_param(gcb,'LinkStatus','inactive')
      | set_param(gcb,'LinkStatus','none')
      | set_param([gcb '/Goto'],'GotoTag', [get(gcbh,'name')])
      | 
      | set_param([gcb '/From'],'GotoTag', [get(gcbh,'name')])
      settings: NameChangeFcn=|
      | set_param([gcb '/Goto'],'GotoTag', [get(gcbh,'name')])
      | 
      | set_param([gcb '/From'],'GotoTag', [get(gcbh,'name')])
      settings: OpenFcn=|
      | open_system([gcb '/ang_vel']);
      | close_system(gcb);                    hh=findobj(allchild(0),'name','ang_vel');
      | ha=findobj(hh(1),'type','axes');
      | set(get(ha,'title'),'string',get(gcbh,'name'));
      | clear hh ha;
      mask Display: port_label('LConn', 1,'W');
  Gear Box : fl_lib/Mechanical/Mechanisms/Gear Box  ratio=Transmission_GearRatio  t_in_Log=off  t_out_Log=off  LocalVarNames=|t_in|t_out  LocalVarDescs=|t_in|t_out  LocalVarLogging=[0 0]
  Inertia1 : fl_lib/Mechanical/Rotational Elements/Inertia  inertia=0.01 kg*m^2  initial_velocity=0 rad/s  t_Log=off  LocalVarNames=|t  LocalVarDescs=|t  LocalVarLogging=0
  Inertia2 : fl_lib/Mechanical/Rotational Elements/Inertia  inertia=0.01 kg*m^2  initial_velocity=0 rad/s  t_Log=off  LocalVarNames=|t  LocalVarDescs=|t  LocalVarLogging=0
  Post-Gear Torque Speed Sensor : Subsystem
      mask Display: disp('Trq N S')
  Pre-Gear Torque Speed Sensor : Subsystem
      mask Display: disp('Trq N S')
  Torque : Subsystem  InitFcn=|
      | unit=get_param([gcb '/PS-S'],'Unit');
      | set_param(gcb, 'AttributesFormatString', strcat('[', unit,']'));
      mask help: Simscape Probe
      settings: AttributesFormatString=[N*m]
      settings: CopyFcn=|
      | set_param(gcb,'LinkStatus','inactive')
      | set_param(gcb,'LinkStatus','none')
      | set_param([gcb '/Goto'],'GotoTag', [get(gcbh,'name')])
      | 
      | set_param([gcb '/From'],'GotoTag', [get(gcbh,'name')])
      settings: NameChangeFcn=|
      | set_param([gcb '/Goto'],'GotoTag', [get(gcbh,'name')])
      | 
      | set_param([gcb '/From'],'GotoTag', [get(gcbh,'name')])
      settings: OpenFcn=|
      | open_system([gcb '/torque']);
      | close_system(gcb);                    hh=findobj(allchild(0),'name','torque');
      | ha=findobj(hh(1),'type','axes');
      | set(get(ha,'title'),'string',get(gcbh,'name'));
      | clear hh ha;
      mask Display:
      | patch([0.5 1 0.5], [0.25 .5 0.75],[0 0 0])
      | plot([0,0.5],[0.5,0.5]);
  Torque1 : Subsystem  InitFcn=|
      | unit=get_param([gcb '/PS-S'],'Unit');
      | set_param(gcb, 'AttributesFormatString', strcat('[', unit,']'));
      mask help: Simscape Probe
      settings: AttributesFormatString=[N*m]
      settings: CopyFcn=|
      | set_param(gcb,'LinkStatus','inactive')
      | set_param(gcb,'LinkStatus','none')
      | set_param([gcb '/Goto'],'GotoTag', [get(gcbh,'name')])
      | 
      | set_param([gcb '/From'],'GotoTag', [get(gcbh,'name')])
      settings: NameChangeFcn=|
      | set_param([gcb '/Goto'],'GotoTag', [get(gcbh,'name')])
      | 
      | set_param([gcb '/From'],'GotoTag', [get(gcbh,'name')])
      settings: OpenFcn=|
      | open_system([gcb '/torque']);
      | close_system(gcb);                    hh=findobj(allchild(0),'name','torque');
      | ha=findobj(hh(1),'type','axes');
      | set(get(ha,'title'),'string',get(gcbh,'name'));
      | clear hh ha;
      mask Display:
      | patch([0.5 1 0.5], [0.25 .5 0.75],[0 0 0])
      | plot([0,0.5],[0.5,0.5]);
  ToFrontWheel : PMIOPort  Port=1  Side=Right
  FromMotor : PMIOPort  Port=2  Side=Left
  connections:
  Post-Gear Torque Speed Sensor/LConn1 -- Gear Box/RConn1
  Inertia1/LConn1 -- FromMotor/RConn1 -- Torque/LConn1
  Torque/RConn1 -- Pre-Gear Torque Speed Sensor/LConn1 -- AngVel1/LConn1
  AngVel/LConn1 -- Post-Gear Torque Speed Sensor/RConn1 -- Torque1/LConn1
  Inertia2/LConn1 -- ToFrontWheel/RConn1 -- Torque1/RConn1
  Pre-Gear Torque Speed Sensor/RConn1 -- Gear Box/LConn1

== system System_HybridMotorcycle_v2/Torque Based Vehicle /Vehicle Body ==
  "Front Tire " : sdl_lib/Tires & Vehicles/Tire (Magic Formula)  parameterization=1  F_z1=3e+3 N  F_x1=3.5e+3 N  kappa1=10  B_m=10  C_m=1.9  D_m=1  E_m=0.97  fz0=4e+3 N  p_Cx=1.685  p_Dx=[ 1.21 -0.037 ]  p_Ex=[ 0.344 0.095 -0.02 0 ]  p_Kx=[ 21.51 -0.163 0.245 ]  p_Hx=[ -0.002 0.002 ]  p_Vx=[ 0 0 ]  v_tr_thr=0.1 m/s  r_e=0.1778 m  model_compliance=0  stiffness=1e+6 N/m  damping=1000 N/(m/s)  model_inertia=0  inertia=1 kg*m^2  initial_velocity=0 rad/s  model_resistance=0  resistance_model=1  coeff=0.015  p_tire=250e3 Pa  alpha=-0.003  beta=0.97  coeff_a=84e-4  coeff_b=6.2e-4 s/m  coeff_c=1.6e-4 s^2/m^2  v_thr=1e-3 m/s  LocalVarLogging=[]
  Rear Tire : sdl_lib/Tires & Vehicles/Tire (Magic Formula)  parameterization=1  F_z1=3e+3 N  F_x1=3.5e+3 N  kappa1=10  B_m=10  C_m=1.9  D_m=1  E_m=0.97  fz0=4e+3 N  p_Cx=1.685  p_Dx=[ 1.21 -0.037 ]  p_Ex=[ 0.344 0.095 -0.02 0 ]  p_Kx=[ 21.51 -0.163 0.245 ]  p_Hx=[ -0.002 0.002 ]  p_Vx=[ 0 0 ]  v_tr_thr=0.1 m/s  r_e=0.1778 m  model_compliance=0  stiffness=1e+6 N/m  damping=1000 N/(m/s)  model_inertia=0  inertia=1 kg*m^2  initial_velocity=0 rad/s  model_resistance=0  resistance_model=1  coeff=0.015  p_tire=250e3 Pa  alpha=-0.003  beta=0.97  coeff_a=84e-4  coeff_b=6.2e-4 s/m  coeff_c=1.6e-4 s^2/m^2  v_thr=1e-3 m/s  LocalVarLogging=[]
  Vehicle Body : sdl_lib/Tires & Vehicles/Vehicle Body  mass=Vehicle_Mass_kg kg  n_w=2  x_f=0.75 m  x_r=0.75 m  y_c=0.5 m  area=Vehicle_FrontalArea_m2 m^2  Cd=Vehicle_DragCoef  v0=0 m/s  g=9.81 m/s^2  rho=1.18 kg/m^3  v_Log=off  f_Log=off  LocalVarNames=|v|f  LocalVarDescs=|v|f  LocalVarLogging=[0 0]
  FromMotorGR : PMIOPort  Port=1  Side=Left
  Conn2 : PMIOPort  Port=2  Side=Right
  FromCVT : PMIOPort  Port=3  Side=Left
  connections:
  "Front Tire "/RConn2 -- Rear Tire/RConn2 -- Vehicle Body/LConn1
  Vehicle Body/RConn1 -- Rear Tire/LConn1
  Vehicle Body/RConn2 -- "Front Tire "/LConn1
  Vehicle Body/LConn2 -- Conn2/RConn1
  FromCVT/RConn1 -- "Front Tire "/LConn2 -- Rear Tire/LConn2

== system System_HybridMotorcycle_v2/Lead Acid Battery Subsystem/Battery cell/ DOC  ==
  PS-Simulink Converter1 : nesl_utility/PS-Simulink Converter  PhysicalDomain=network_engine_domain  SubClassName=ps_output  LeftPortType=input  RightPortType=output  PseudoPeriodic=off  Frequencies=[]  Unit=1  AffineConversion=off
  PS : PMIOPort  Port=1  Side=Left
  tag scope: DOC=global
  wires:
  PS-Simulink Converter1/1 -> [DOC]
  connections:
  PS/RConn1 -- PS-Simulink Converter1/LConn1

== system System_HybridMotorcycle_v2/Lead Acid Battery Subsystem/Battery cell/ SOC  ==
  PS-Simulink Converter1 : nesl_utility/PS-Simulink Converter  PhysicalDomain=network_engine_domain  SubClassName=ps_output  LeftPortType=input  RightPortType=output  PseudoPeriodic=off  Frequencies=[]  Unit=1  AffineConversion=off
  PS : PMIOPort  Port=1  Side=Left
  tag scope: SOC=global
  wires:
  PS-Simulink Converter1/1 -> [SOC]
  connections:
  PS/RConn1 -- PS-Simulink Converter1/LConn1

== system System_HybridMotorcycle_v2/Lead Acid Battery Subsystem/Battery cell/T ==
  PS-Simulink Converter1 : nesl_utility/PS-Simulink Converter  PhysicalDomain=network_engine_domain  SubClassName=ps_output  LeftPortType=input  RightPortType=output  PseudoPeriodic=off  Frequencies=[]  Unit=C  AffineConversion=on
  PS : PMIOPort  Port=1  Side=Left
  tag scope: T=global
  wires:
  PS-Simulink Converter1/1 -> [T]
  connections:
  PS/RConn1 -- PS-Simulink Converter1/LConn1

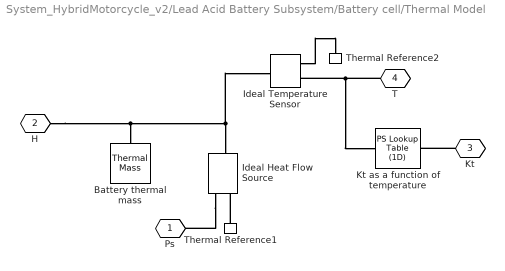
== system System_HybridMotorcycle_v2/Lead Acid Battery Subsystem/Battery cell/Thermal Model ==
  Battery thermal mass : fl_lib/Thermal/Thermal Elements/Thermal Mass  mass=1 kg  sp_heat=Ctheta J/kg/K  init_temp=theta_init+273 K  Q_Log=off  LocalVarNames=|heat_flow|temperature  LocalVarDescs=|Heat flow (J/s)|Mass temperature (K)  LocalVarLogging=[0 0]
  Ideal Temperature Sensor : fl_lib/Thermal/Thermal Sensors/Ideal Temperature Sensor  Qs_Log=off  Ts_Log=off  LocalVarNames=|Qs|Ts  LocalVarDescs=|Qs|Ts  LocalVarLogging=[]
  Ideal Heat Flow Source : fl_lib/Thermal/Thermal Sources/Ideal Heat Flow Source  Q_Log=off  T_Log=off  LocalVarNames=|heat_flow|T_differential  LocalVarDescs=|Heat flow through the source (J/s)|Temperature differential across the source (K)  LocalVarLogging=[0 0]
  Kt as a function of temperature : fl_lib/Physical Signals/Lookup Tables/PS Lookup Table (1D)  x_t=[theta_f, Kt_Temps]+273  y_t=[0 Kt]  interp_method=1  extrap_method=1  LocalVarLogging=[]
  Thermal Reference1 : fl_lib/Thermal/Thermal Elements/Thermal Reference  Q_Log=off  LocalVarNames=|Q  LocalVarDescs=|Q  LocalVarLogging=[]
  Thermal Reference2 : fl_lib/Thermal/Thermal Elements/Thermal Reference  Q_Log=off  LocalVarNames=|Q  LocalVarDescs=|Q  LocalVarLogging=[]
  Ps : PMIOPort  Tag=PMCPort  Port=1  Side=Left
  H : PMIOPort  Tag=PMCPort  Port=2  Side=Left
  Kt : PMIOPort  Tag=PMCPort  Port=3  Side=Right
  T : PMIOPort  Tag=PMCPort  Port=4  Side=Right
  connections:
  Ideal Temperature Sensor/RConn1 -- Thermal Reference2/LConn1
  Ideal Temperature Sensor/RConn2 -- Kt as a function of temperature/LConn1 -- T/RConn1
  Thermal Reference1/LConn1 -- Ideal Heat Flow Source/RConn2
  H/RConn1 -- Ideal Temperature Sensor/LConn1 -- Ideal Heat Flow Source/LConn1 -- Battery thermal mass/LConn1
  Kt/RConn1 -- Kt as a function of temperature/RConn1
  Ideal Heat Flow Source/RConn1 -- Ps/RConn1
